simulink model "zygo_demo_position"  (Simulink 7.4)
settings: Solver=FixedStepDiscrete  StartTime=0.0  StopTime=inf  FixedStep=0.001  RelTol=1e-3
libraries: xpclib x4, speedgoatlib_ZMI4104 x4
settings Model: Creator=dkuratli  LastModifiedBy=lab3  BufferReuse=off
settings OptimizationCC: BlockReduction=off  OptimizeBlockIOStorage=off  BufferReuse=off  ExpressionFolding=off  LocalBlockOutputs=off
settings DebuggingCC: FcnCallInpInsideContextMsg=Enable All  StrictBusMsg=ErrorLevel1
settings HardwareCC: ProdIntDivRoundTo=Zero  ProdEndianess=LittleEndian  ProdHWDeviceType=Generic->32-bit x86 compatible
settings RTWCC: SystemTargetFile=xpctarget.tlc  TemplateMakefile=xpc_default_tmf  Description=Simulink Real-Time  ProcessScript=xpctarget_make_rtw_hook  RTWCompilerOptimization=On
settings CodeAppCC: CustomSymbolStrType=$N$R$M_T
settings xpcTargetCC: TargetFcnLib=ansi_tfl_table_tmw.mat  TargetFunctionLibrary=ANSI_C  ParMdlRefBuildCompliant=on  ConcurrentExecutionCompliant=on  CombineSignalStateStructs=off  GRTInterface=on  GenerateAllocFcn=off  xPCTaskExecutionProfile=off  xPCRL32EventNumber=5000  xPCisModelTimeout=off  xPCModelTimeoutSecs=15  xPCLoadParamSetFile=off  xPCConcurrentTasks=off  xPCEnableSFAnimation=off

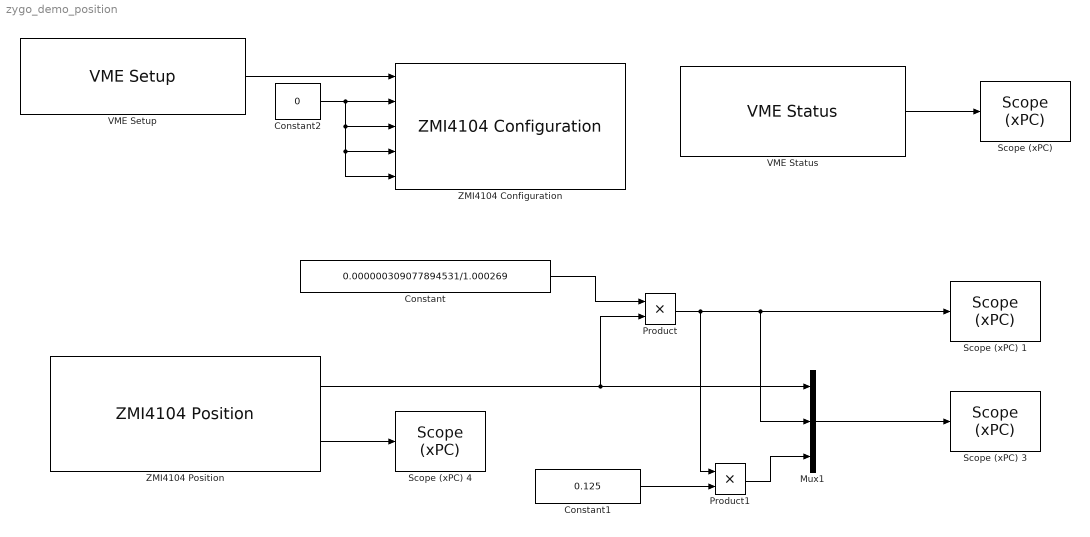
== system zygo_demo_position ==
  Constant : Constant  Value=0.000000309077894531/1.000269
  Constant1 : Constant  Value=0.125
  Constant2 : Constant  Value=0
  Mux1 : Mux  Inputs=3
  Product : Product  RndMeth=Zero
  Product1 : Product  RndMeth=Zero
  "Scope (xPC) " : xpclib/Misc./Scope (xPC)   scopeno=1  scopetype=Target  autostart=on  viewmode=Numerical  formatstr='VME link error: %1.0f'  grid=on  ylimits=[0,0]  nosamples=3  noprepostsamples=0  interleave=1  triggermode=FreeRun  triggersignal=1  trigsignalfromport=off  triggerlevel=0.0  triggerslope=Either  triggerscope=1  triggersample=0  filename=data.dat  mode=Lazy  writesize=512  autorestart=off  dynamicfilemode=off  maxwritefilesize=512*1024^2
  Scope (xPC) 1 : xpclib/Misc./Scope (xPC)   scopeno=4  scopetype=Target  autostart=on  viewmode=Graphical redraw  formatstr='Time: %15.6f'  grid=on  ylimits=[0,0]  nosamples=250  noprepostsamples=0  interleave=1  triggermode=FreeRun  triggersignal=1  trigsignalfromport=off  triggerlevel=0.0  triggerslope=Either  triggerscope=1  triggersample=0  filename=data.dat  mode=Lazy  writesize=512  autorestart=off  dynamicfilemode=off  maxwritefilesize=512*1024^2
  Scope (xPC) 3 : xpclib/Misc./Scope (xPC)   scopeno=2  scopetype=Target  autostart=on  viewmode=Numerical  formatstr='Register value: %f,With your factor: %f,With 0.125 factor: %f'  grid=on  ylimits=[0,0]  nosamples=10  noprepostsamples=0  interleave=1  triggermode=FreeRun  triggersignal=1  trigsignalfromport=off  triggerlevel=0.0  triggerslope=Either  triggerscope=1  triggersample=0  filename=data.dat  mode=Lazy  writesize=512  autorestart=off  dynamicfilemode=off  maxwritefilesize=512*1024^2
  Scope (xPC) 4 : xpclib/Misc./Scope (xPC)   scopeno=3  scopetype=Target  autostart=on  viewmode=Numerical  formatstr='Time: %15.6f'  grid=on  ylimits=[0,0]  nosamples=3  noprepostsamples=0  interleave=1  triggermode=FreeRun  triggersignal=1  trigsignalfromport=off  triggerlevel=0.0  triggerslope=Either  triggerscope=1  triggersample=0  filename=data.dat  mode=Lazy  writesize=512  autorestart=off  dynamicfilemode=off  maxwritefilesize=512*1024^2
  VME Setup : speedgoatlib_ZMI4104/VME Setup  id=1  modules=1  slot=-1  z1_id=1  z1_addr_sw1=0  z1_addr_sw2=0  z2_id=2  z2_addr_sw1=0  z2_addr_sw2=1
  VME Status : speedgoatlib_ZMI4104/VME Status  id=1  ts=-1  slot=-1
  ZMI4104 Configuration : speedgoatlib_ZMI4104/ZMI4104 Configuration  id=1  ts=-1  slot=-1  ax1_filter_kv=-19  ax1_filter_kp=-8  ax2_filter_kv=-19  ax2_filter_kp=-8  ax3_filter_kv=-19  ax3_filter_kp=-8  ax4_filter_kv=-19  ax4_filter_kp=-8
  ZMI4104 Position : speedgoatlib_ZMI4104/ZMI4104 Position  id=1  zmi_id=1  axis=1  ts=-1  slot=-1  act_vel=off  act_time=on
  wires:
  VME Setup/1 -> ZMI4104 Configuration/1
  Constant2/1 -> ZMI4104 Configuration/2, ZMI4104 Configuration/5, ZMI4104 Configuration/4, ZMI4104 Configuration/3
  VME Status/1 -> "Scope (xPC) "/1
  ZMI4104 Position/1 -> Product/2, Mux1/1
  Constant/1 -> Product/1
  Mux1/1 -> Scope (xPC) 3/1
  Product/1 -> Product1/1, Mux1/2, Scope (xPC) 1/1
  Constant1/1 -> Product1/2
  Product1/1 -> Mux1/3
  ZMI4104 Position/2 -> Scope (xPC) 4/1
